simulink model "GENMODEL"  (Simulink 7.3)
settings: Solver=ode45  StartTime=0.0  StopTime=10.0  RelTol=1e-3
settings Model: Creator=leela  LastModifiedBy=P.R.BHANUTEJA

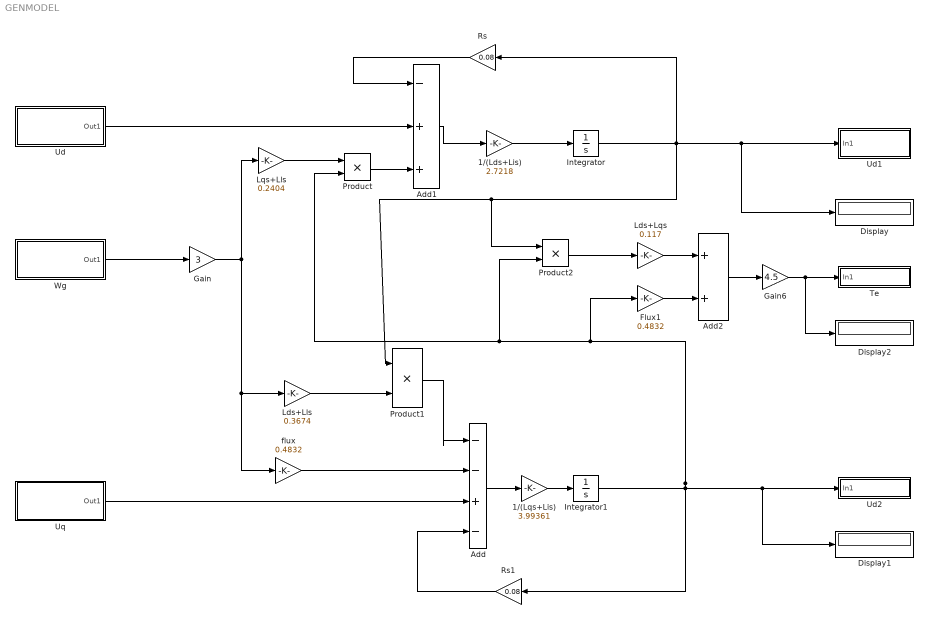
== system GENMODEL ==
  1/(Lds+Lis) : Gain  Gain=2.7218  ParameterDataType=fixdt(1, 16)  ParameterScaling=2^0  OutDataType=fixdt(1, 16)  OutScaling=2^0
  1/(Lqs+Lis) : Gain  Gain=3.99361  ParameterDataType=fixdt(1, 16)  ParameterScaling=2^0  OutDataType=fixdt(1, 16)  OutScaling=2^0
  Add : Sum  Inputs=--+-  OutDataType=fixdt(1, 16)  OutScaling=2^-10
  Add1 : Sum  Inputs=-++  OutDataType=fixdt(1, 16)  OutScaling=2^-10
  Add2 : Sum  OutDataType=fixdt(1, 16)  OutScaling=2^-10
  Display : Display
  Display1 : Display
  Display2 : Display
  Flux1 : Gain  Gain=0.4832  ParameterDataType=fixdt(1, 16)  ParameterScaling=2^0  OutDataType=fixdt(1, 16)  OutScaling=2^0
  Gain : Gain  Gain=3  ParameterDataType=fixdt(1, 16)  ParameterScaling=2^0  OutDataType=fixdt(1, 16)  OutScaling=2^0
  Gain6 : Gain  Gain=4.5  ParameterDataType=fixdt(1, 16)  ParameterScaling=2^0  OutDataType=fixdt(1, 16)  OutScaling=2^0
  Integrator : Integrator
  Integrator1 : Integrator
  Lds+Lls : Gain  Gain=0.3674  ParameterDataType=fixdt(1, 16)  ParameterScaling=2^0  OutDataType=fixdt(1, 16)  OutScaling=2^0
  Lds+Lqs : Gain  Gain=0.117  ParameterDataType=fixdt(1, 16)  ParameterScaling=2^0  OutDataType=fixdt(1, 16)  OutScaling=2^0
  Lqs+Lls : Gain  Gain=0.2404  ParameterDataType=fixdt(1, 16)  ParameterScaling=2^0  OutDataType=fixdt(1, 16)  OutScaling=2^0
  Product : Product  OutDataType=fixdt(1, 16)  OutScaling=2^0  RndMeth=Zero
  Product1 : Product  OutDataType=fixdt(1, 16)  OutScaling=2^0  RndMeth=Zero
  Product2 : Product  OutDataType=fixdt(1, 16)  OutScaling=2^0  RndMeth=Zero
  Rs : Gain  Gain=0.08  ParameterDataType=fixdt(1, 16)  ParameterScaling=2^0  OutDataType=fixdt(1, 16)  OutScaling=2^0
  Rs1 : Gain  Gain=0.08  ParameterDataType=fixdt(1, 16)  ParameterScaling=2^0  OutDataType=fixdt(1, 16)  OutScaling=2^0
  Te : Subsystem  TreatAsAtomicUnit=on
  Ud : Subsystem  TreatAsAtomicUnit=on
  Ud1 : Subsystem  TreatAsAtomicUnit=on
  Ud2 : Subsystem  TreatAsAtomicUnit=on
  Uq : Subsystem  TreatAsAtomicUnit=on
  Wg : Subsystem  TreatAsAtomicUnit=on
  flux : Gain  Gain=0.4832  ParameterDataType=fixdt(1, 16)  ParameterScaling=2^0  OutDataType=fixdt(1, 16)  OutScaling=2^0
  wires:
  Wg/1(Out1) -> Gain/1
  Lqs+Lls/1 -> Product/1
  Gain/1 -> Lqs+Lls/1, Lds+Lls/1, flux/1
  Product/1 -> Add1/3
  Ud/1(Out1) -> Add1/2
  Rs/1 -> Add1/1
  Add1/1 -> 1/(Lds+Lis)/1
  1/(Lds+Lis)/1 -> Integrator/1
  Integrator/1 -> Ud1/1(In1), Display/1, Rs/1, Product1/1, Product2/1
  Lds+Lls/1 -> Product1/2
  Product2/1 -> Lds+Lqs/1
  Integrator1/1 -> Flux1/1, Product/2, Product2/2, Rs1/1, Ud2/1(In1), Display1/1
  Flux1/1 -> Add2/2
  Lds+Lqs/1 -> Add2/1
  Add2/1 -> Gain6/1
  Gain6/1 -> Te/1(In1), Display2/1
  Product1/1 -> Add/1
  flux/1 -> Add/2
  Uq/1(Out1) -> Add/3
  1/(Lqs+Lis)/1 -> Integrator1/1
  Add/1 -> 1/(Lqs+Lis)/1
  Rs1/1 -> Add/4

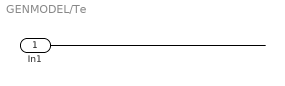
== system GENMODEL/Te ==
  In1 : Inport  OutDataType=fixdt(1, 16)  OutScaling=2^0
  wires:
  In1/1 -> ?

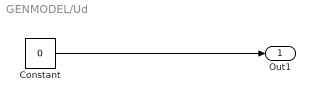
== system GENMODEL/Ud ==
  Constant : Constant  Value=0  OutDataType=fixdt(1, 16)  OutScaling=2^0
  Out1 : Outport  OutDataType=fixdt(1, 16)  OutScaling=2^0
  wires:
  Constant/1 -> Out1/1

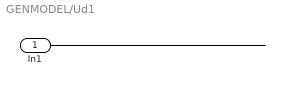
== system GENMODEL/Ud1 ==
  In1 : Inport  OutDataType=fixdt(1, 16)  OutScaling=2^0
  wires:
  In1/1 -> ?

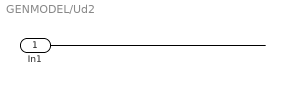
== system GENMODEL/Ud2 ==
  In1 : Inport  OutDataType=fixdt(1, 16)  OutScaling=2^0
  wires:
  In1/1 -> ?

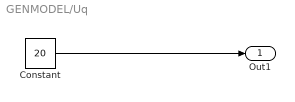
== system GENMODEL/Uq ==
  Constant : Constant  Value=20  OutDataType=fixdt(1, 16)  OutScaling=2^0
  Out1 : Outport  OutDataType=fixdt(1, 16)  OutScaling=2^0
  wires:
  Constant/1 -> Out1/1

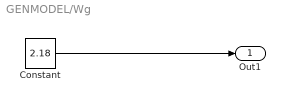
== system GENMODEL/Wg ==
  Constant : Constant  Value=2.18  OutDataType=fixdt(1, 16)  OutScaling=2^0
  Out1 : Outport  OutDataType=fixdt(1, 16)  OutScaling=2^0
  wires:
  Constant/1 -> Out1/1
